simulink model "steady_state_model_verification"  (R2022b)
settings: Solver=VariableStepAuto  StartTime=0.0  StopTime=tmax  FixedStep=sample_time/10  RelTol=1e-3
values from neighbouring files (symbols this model uses):
  D = D_amp * exp(1i * angle(V_required))    [custom_control.m]    (also in steady_state_model_verification_script.m = D_amp .* exp(1i*D_phase))
  driving_voltage = 48    [sim_params.m]
  k = 0.1    [sim_params.m]    (also in steady_state_model_verification_script.m = k_vals(i))
  max_current = 150    [sim_params.m]
  phase_nbits = 16    [sim_params.m]
  R1 = 0.26    [sim_params.m]
  R2 = 0.26    [sim_params.m]
  relative_deadtime = deadtime / (0.5/fc)    (= 0.2164375)    [sim_params.m]
  sample_time = 1/(fc*samples_per_period)    (= 2.25599191452e-07)    [sim_params.m]
  samples_per_period = 32*4    (= 128)    [sim_params.m]
libraries: simulink x10, fl_lib x6, nesl_utility x5, ee_lib x4
settings Model: Creator=knasr  LastModifiedBy=nasrk
settings DebuggingCC: ParameterPrecisionLossMsg=none

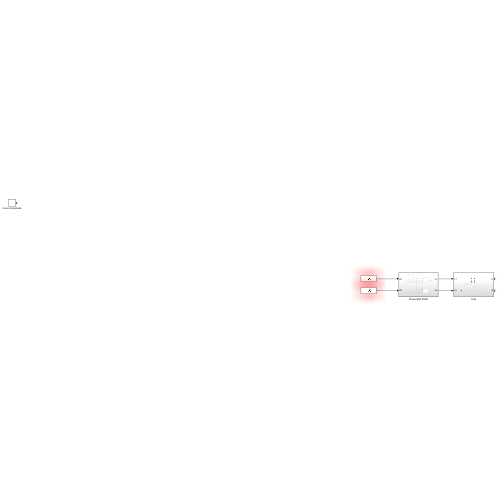
[thumbnail: Simulink's stored preview of the top-level diagram]
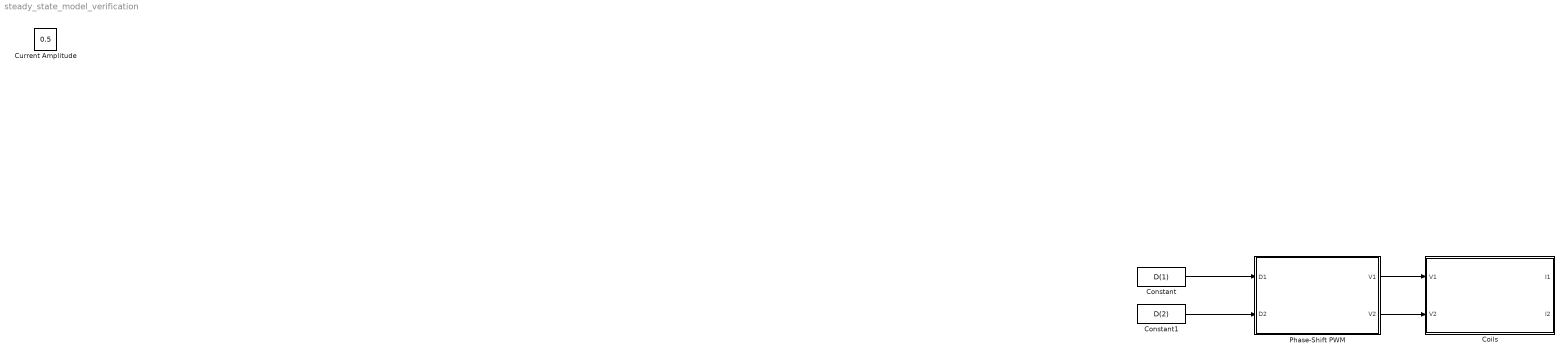
== system steady_state_model_verification ==
  Coils : Subsystem
  Constant : Constant  Value=D(1)  SampleTime=sample_time
  Constant1 : Constant  Value=D(2)  SampleTime=sample_time
  Current Amplitude : Constant  Value=0.5
  Phase-Shift PWM : Subsystem
  wires:
  Phase-Shift PWM/1(V1) -> Coils/1(V1)
  Phase-Shift PWM/2(V2) -> Coils/2(V2)
  Constant/1 -> Phase-Shift PWM/1(D1)
  Constant1/1 -> Phase-Shift PWM/2(D2)

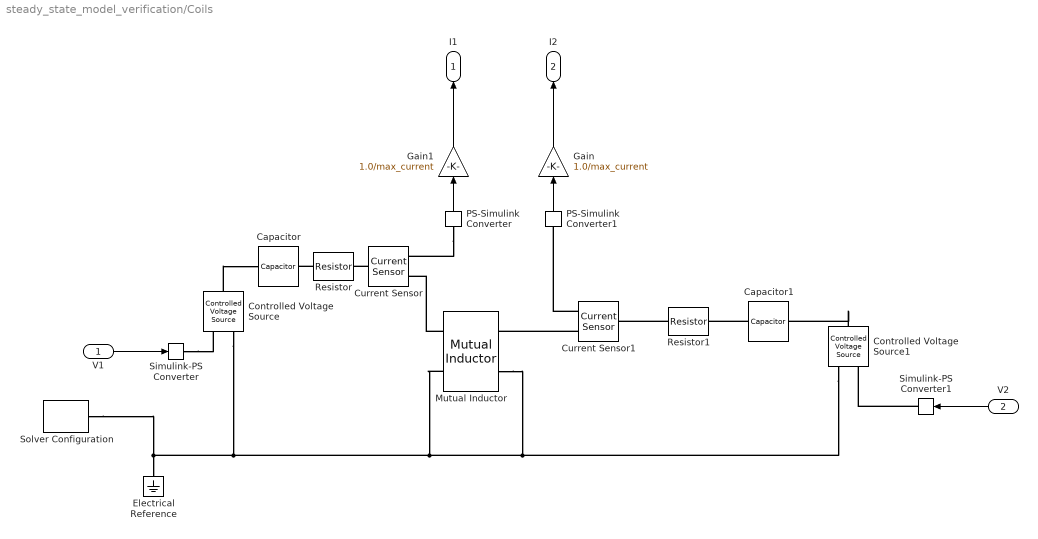
== system steady_state_model_verification/Coils ==
  V1 : Inport
  V2 : Inport  Port=2
  Capacitor : ee_lib/Passive/Capacitor  cap_option=0  c=C1 F  Cvec=[1e-05, 1e-06] F  Vvec=[0, 10] V  CV_table_symmetry=1  f_vec=[1, 10] kHz  DFext_vec=[.8, 1.2]  enable_C_tol=0  C_tol=5  tol_distribution=1  nSigma=4  r=1e-6 Ohm  g=0 1/Ohm  averaging_period=0 s  enable_operating_limits=0  operating_limit_action=2  max_working_voltage_range=[-25, 25] V  power_rating=1 W  enable_faults=0  fault_action=1  Cscale_faulted=100  R_faulted=1e-3 Ohm  G_faulted=0 1/Ohm  tau_fault=1e-3 s  enable_temporal_fault=0  t_fault=1 s  enable_behavioral_fault=0  max_permissible_voltage_range=[-100, 100] V  t_fail_on_voltage=1 s  i_specify=off  i_priority=None  i=0 A  i_nominal_specify=off  i_nominal_unit=A  i_nominal_value=1  v_specify=off  v_priority=None  v=0 V  v_nominal_specify=off  v_nominal_unit=V  v_nominal_value=1  vc_specify=off  vc_priority=High  vc=0 V  vc_nominal_specify=off  vc_nominal_unit=V  vc_nominal_value=1
  Capacitor1 : ee_lib/Passive/Capacitor  cap_option=0  c=C2 F  Cvec=[1e-05, 1e-06] F  Vvec=[0, 10] V  CV_table_symmetry=1  f_vec=[1, 10] kHz  DFext_vec=[.8, 1.2]  enable_C_tol=0  C_tol=5  tol_distribution=1  nSigma=4  r=1e-6 Ohm  g=0 1/Ohm  averaging_period=0 s  enable_operating_limits=0  operating_limit_action=2  max_working_voltage_range=[-25, 25] V  power_rating=1 W  enable_faults=0  fault_action=1  Cscale_faulted=100  R_faulted=1e-3 Ohm  G_faulted=0 1/Ohm  tau_fault=1e-3 s  enable_temporal_fault=0  t_fault=1 s  enable_behavioral_fault=0  max_permissible_voltage_range=[-100, 100] V  t_fail_on_voltage=1 s  i_specify=off  i_priority=None  i=0 A  i_nominal_specify=off  i_nominal_unit=A  i_nominal_value=1  v_specify=off  v_priority=None  v=0 V  v_nominal_specify=off  v_nominal_unit=V  v_nominal_value=1  vc_specify=off  vc_priority=High  vc=0 V  vc_nominal_specify=off  vc_nominal_unit=V  vc_nominal_value=1
  Controlled Voltage Source : fl_lib/Electrical/Electrical Sources/Controlled Voltage Source
  Controlled Voltage Source1 : fl_lib/Electrical/Electrical Sources/Controlled Voltage Source
  Current Sensor : fl_lib/Electrical/Electrical Sensors/Current Sensor
  Current Sensor1 : fl_lib/Electrical/Electrical Sensors/Current Sensor
  Electrical Reference : fl_lib/Electrical/Electrical Elements/Electrical Reference
  Gain : Gain  Gain=1.0/max_current
  Gain1 : Gain  Gain=1.0/max_current
  Mutual Inductor : fl_lib/Electrical/Electrical Elements/Mutual Inductor  L1=L1 H  L2=L2 H  k=k  i1_specify=off  i1_priority=High  i1=0 A  i1_nominal_specify=off  i1_nominal_unit=A  i1_nominal_value=1  i2_specify=off  i2_priority=High  i2=0 A  i2_nominal_specify=off  i2_nominal_unit=A  i2_nominal_value=1  v1_specify=off  v1_priority=None  v1=0 V  v1_nominal_specify=off  v1_nominal_unit=V  v1_nominal_value=1  v2_specify=off  v2_priority=None  v2=0 V  v2_nominal_specify=off  v2_nominal_unit=V  v2_nominal_value=1
      settings: InternalSimscapePortConfiguration="{\"Bottom\":[],\"Left\":[{\"id\":\"p1\",\"label\":\"1+\",\"type\":\"foundation.electrical.electrical\"},{\"id\":\"n1\",\"label\":\"1-\",\"type\":\"foundation.electrical.electrical\"}],\"Right\":[{\"id\":\"p2\",\"label\":\"2+\",\"type\":\"foundation.electrical.electrical\"},{\"id\":\"n2\",\"label\":\"2-\",\"type\":\"foundation.electrical.electrical\"}],\"Top\":[]}"
  PS-Simulink Converter : nesl_utility/PS-Simulink Converter  PhysicalDomain=network_engine_domain  SubClassName=ps_output  LeftPortType=input  RightPortType=output  PseudoPeriodic=off  Frequencies=[]  VectorFormat=inherit  Unit=inherit  AffineConversion=off
  PS-Simulink Converter1 : nesl_utility/PS-Simulink Converter  PhysicalDomain=network_engine_domain  SubClassName=ps_output  LeftPortType=input  RightPortType=output  PseudoPeriodic=off  Frequencies=[]  VectorFormat=inherit  Unit=inherit  AffineConversion=off
  Resistor : ee_lib/Passive/Resistor  R=R1 Ohm  enable_R_tol=0  R_tol=5  tol_distribution=1  nSigma=4  enable_operating_limits=0  operating_limit_action=2  max_working_voltage=100 V  power_rating=1 W  enable_faults=0  fault_action=1  R_faulted=inf Ohm  enable_temporal_fault=0  t_fault=1 s  enable_behavioral_fault=0  max_permissible_current=1 A  t_fail_on_current=1 s  noise_mode=0  sample_time=1e-3 s  repeatability=1  auto_seed=545404223  user_seed=0  Tdevice=25 degC  power_derating_T1=70 degC  power_derating_T2=155 degC  operating_temperature_range_vec=[-50, 150] degC  alpha=3.93e-3 1/K  Tmeas=25 degC  thermal_mass=100 J/K  temperature_specify=off  temperature_priority=High  temperature=298.15 K  temperature_nominal_specify=off  temperature_nominal_unit=K  temperature_nominal_value=1
  Resistor1 : ee_lib/Passive/Resistor  R=R2 Ohm  enable_R_tol=0  R_tol=5  tol_distribution=1  nSigma=4  enable_operating_limits=0  operating_limit_action=2  max_working_voltage=100 V  power_rating=1 W  enable_faults=0  fault_action=1  R_faulted=inf Ohm  enable_temporal_fault=0  t_fault=1 s  enable_behavioral_fault=0  max_permissible_current=1 A  t_fail_on_current=1 s  noise_mode=0  sample_time=1e-3 s  repeatability=1  auto_seed=3922919431  user_seed=0  Tdevice=25 degC  power_derating_T1=70 degC  power_derating_T2=155 degC  operating_temperature_range_vec=[-50, 150] degC  alpha=3.93e-3 1/K  Tmeas=25 degC  thermal_mass=100 J/K  temperature_specify=off  temperature_priority=High  temperature=298.15 K  temperature_nominal_specify=off  temperature_nominal_unit=K  temperature_nominal_value=1
  Simulink-PS Converter : nesl_utility/Simulink-PS Converter  PhysicalDomain=network_engine_domain  SubClassName=ps_input  LeftPortType=input  RightPortType=output  PseudoPeriodic=off  Frequencies=[]  NoiseDistribution=none  NoiseParameters=[]  Unit=1  AffineConversion=off  FilteringAndDerivatives=provide  SimscapeFilterOrder=1  InputFilterTimeConstant=0.001  UdotUserProvided=0
  Simulink-PS Converter1 : nesl_utility/Simulink-PS Converter  PhysicalDomain=network_engine_domain  SubClassName=ps_input  LeftPortType=input  RightPortType=output  PseudoPeriodic=off  Frequencies=[]  NoiseDistribution=none  NoiseParameters=[]  Unit=1  AffineConversion=off  FilteringAndDerivatives=provide  SimscapeFilterOrder=1  InputFilterTimeConstant=0.001  UdotUserProvided=0
  Solver Configuration : nesl_utility/Solver Configuration  PhysicalDomain=network_engine_domain  SubClassName=solver  LeftPortType=input  RightPortType=generic  Tones=[]  Harmonics=[]  SimulateNoise=off  Profile=off  UseLocalSampling=off  EnableSwitchedLinearOptims=on  FrequencyDomain=off  UseCCode=off  RelTol=0.001  AbsTol=1e-06  MinStep=1e-09  ToWorkspace=off  RevertToSquareIcSolve=off  NumHomotopyIterations=100  PhasorMode=off  PhasorModeNumHarmonics=1  ConsistencySolver=NEWTON_XTOL_AFTER_FTOL  IndexReductionMethod=DerivativeReplacement  DoDC=off  ResidualTolerance=1e-09  ConsistencyTolSource=GLOBAL  ConsistencyAbsTol=0.001  ConsistencyRelTol=0.001  ConsistencyTolFactor=0.001  UseLocalSolver=off  LocalSolverChoice=NE_BACKWARD_EULER_ADVANCER  ResolveIndetEquations=on  FunctionEvalNumThread=1  LocalSolverSampleTime=0.001  DoFixedCost=off  MaxNonlinIter=3  MaxModeIter=2  ComputeImpulses=off  ImpulseIterations=2  LinearAlgebra=auto  LinearAlgebraNumThread=0  EquationFormulation=NE_TIME_EF  DelaysMemoryBudget=1024  AutomaticFiltering=on  FilteringTimeConstant=0.001  PartitionStorageMethod=AS_NEEDED  PartitionMemoryBudget=1024  PartitionMethod=ROBUST
  I1 : Outport
  I2 : Outport  Port=2
  wires:
  V1/1 -> Simulink-PS Converter/1
  PS-Simulink Converter/1 -> Gain1/1
  V2/1 -> Simulink-PS Converter1/1
  PS-Simulink Converter1/1 -> Gain/1
  Gain/1 -> I2/1
  Gain1/1 -> I1/1
  connections:
  Mutual Inductor/RConn2 -- Mutual Inductor/LConn2 -- Solver Configuration/RConn1 -- Electrical Reference/LConn1 -- Controlled Voltage Source/RConn2 -- Controlled Voltage Source1/RConn2
  Resistor/LConn1 -- Capacitor/LConn1
  Current Sensor/LConn1 -- Resistor/RConn1
  Simulink-PS Converter/RConn1 -- Controlled Voltage Source/RConn1
  PS-Simulink Converter/LConn1 -- Current Sensor/RConn1
  Controlled Voltage Source/LConn1 -- Capacitor/RConn1
  Mutual Inductor/LConn1 -- Current Sensor/RConn2
  Capacitor1/RConn1 -- Resistor1/RConn1
  Simulink-PS Converter1/RConn1 -- Controlled Voltage Source1/RConn1
  Controlled Voltage Source1/LConn1 -- Capacitor1/LConn1
  Resistor1/LConn1 -- Current Sensor1/LConn1
  Current Sensor1/RConn2 -- Mutual Inductor/RConn1
  Current Sensor1/RConn1 -- PS-Simulink Converter1/LConn1

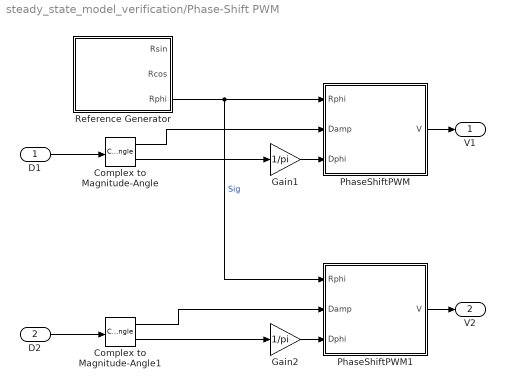
== system steady_state_model_verification/Phase-Shift PWM ==
  D1 : Inport
  D2 : Inport  Port=2
  Complex to Magnitude-Angle : ComplexToMagnitudeAngle
  Complex to Magnitude-Angle1 : ComplexToMagnitudeAngle
  Gain1 : Gain  Gain=1/pi
  Gain2 : Gain  Gain=1/pi
  PhaseShiftPWM : Subsystem
  PhaseShiftPWM1 : Subsystem
  Reference Generator : Subsystem
  V1 : Outport
  V2 : Outport  Port=2
  wires:
  D2/1 -> Complex to Magnitude-Angle1/1
  Complex to Magnitude-Angle/2 -> Gain1/1
  Complex to Magnitude-Angle1/2 -> Gain2/1
  Complex to Magnitude-Angle1/1 -> PhaseShiftPWM1/2(Damp)
  D1/1 -> Complex to Magnitude-Angle/1
  Gain1/1 -> PhaseShiftPWM/3(Dphi)
  Gain2/1 -> PhaseShiftPWM1/3(Dphi)
  Reference Generator/3(Rphi) -> PhaseShiftPWM1/1(Rphi), PhaseShiftPWM/1(Rphi)  "Sig"
  Complex to Magnitude-Angle/1 -> PhaseShiftPWM/2(Damp)
  PhaseShiftPWM/1(V) -> V1/1
  PhaseShiftPWM1/1(V) -> V2/1

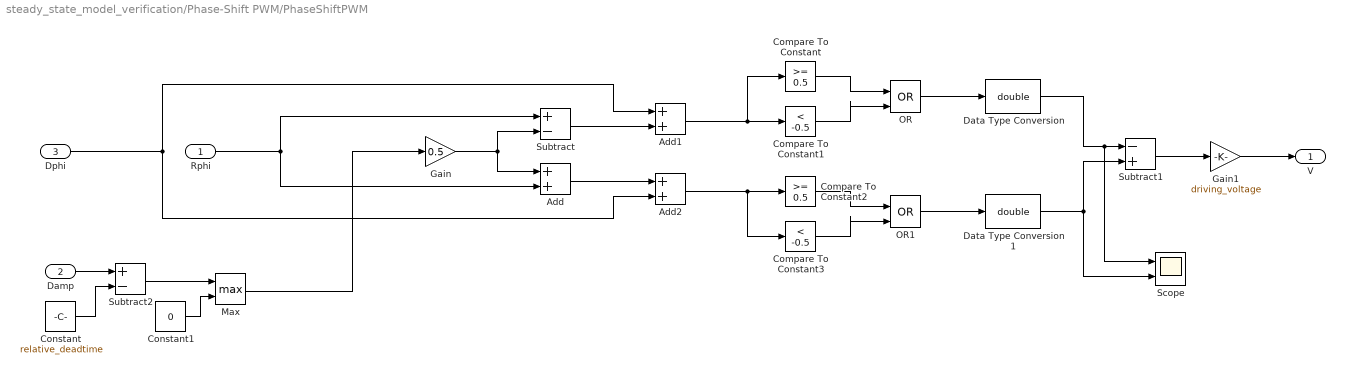
== system steady_state_model_verification/Phase-Shift PWM/PhaseShiftPWM ==
  Rphi : Inport
  Damp : Inport  Port=2
  Dphi : Inport  Port=3
  Add : Sum  AccumDataTypeStr=fixdt(1,phase_nbits,phase_nbits-1)  OutDataTypeStr=fixdt(1,phase_nbits,phase_nbits-1)
  Add1 : Sum  AccumDataTypeStr=fixdt(1,phase_nbits,phase_nbits-1)  OutDataTypeStr=fixdt(1,phase_nbits,phase_nbits-1)
  Add2 : Sum  AccumDataTypeStr=fixdt(1,phase_nbits,phase_nbits-1)  OutDataTypeStr=fixdt(1,phase_nbits,phase_nbits-1)
  Compare To Constant : simulink/Logic and Bit Operations/Compare To Constant  relop=>=  const=0.5  OutDataTypeStr=boolean
  Compare To Constant1 : simulink/Logic and Bit Operations/Compare To Constant  relop=<  const=-0.5  OutDataTypeStr=boolean
  Compare To Constant2 : simulink/Logic and Bit Operations/Compare To Constant  relop=>=  const=0.5  OutDataTypeStr=boolean
  Compare To Constant3 : simulink/Logic and Bit Operations/Compare To Constant  relop=<  const=-0.5  OutDataTypeStr=boolean
  Constant : Constant  Value=relative_deadtime
  Constant1 : Constant  Value=0
  Data Type Conversion : DataTypeConversion  OutDataTypeStr=double  SaturateOnIntegerOverflow=off  RndMeth=Floor
  Data Type Conversion1 : DataTypeConversion  OutDataTypeStr=double  SaturateOnIntegerOverflow=off  RndMeth=Floor
  Gain : Gain  Gain=0.5  ParamDataTypeStr=fixdt(1,phase_nbits,phase_nbits-1)  OutDataTypeStr=fixdt(1,phase_nbits,phase_nbits-1)
  Gain1 : Gain  Gain=driving_voltage
  Max : MinMax  Function=max  Inputs=2
  OR : Logic  Operator=OR  IconShape=distinctive  AllPortsSameDT=off  OutDataTypeStr=boolean
  OR1 : Logic  Operator=OR  IconShape=distinctive  AllPortsSameDT=off  OutDataTypeStr=boolean
  Scope : Scope  NumInputPorts=2
  Subtract : Sum  Inputs=+-  AccumDataTypeStr=fixdt(1,phase_nbits,phase_nbits-1)  OutDataTypeStr=fixdt(1,phase_nbits,phase_nbits-1)
  Subtract1 : Sum  Inputs=-+
  Subtract2 : Sum  Inputs=+-
  V : Outport
  wires:
  Gain/1 -> Add/1, Subtract/2
  Rphi/1 -> Subtract/1, Add/2
  Subtract/1 -> Add1/2
  Add/1 -> Add2/1
  Dphi/1 -> Add1/1, Add2/2
  Add1/1 -> Compare To Constant/1, Compare To Constant1/1
  Compare To Constant/1 -> OR/1
  Compare To Constant1/1 -> OR/2
  Compare To Constant2/1 -> OR1/1
  Compare To Constant3/1 -> OR1/2
  Add2/1 -> Compare To Constant3/1, Compare To Constant2/1
  OR1/1 -> Data Type Conversion1/1
  OR/1 -> Data Type Conversion/1
  Data Type Conversion/1 -> Scope/1, Subtract1/1
  Data Type Conversion1/1 -> Subtract1/2, Scope/2
  Subtract1/1 -> Gain1/1
  Gain1/1 -> V/1
  Damp/1 -> Subtract2/1
  Constant/1 -> Subtract2/2
  Subtract2/1 -> Max/1
  Constant1/1 -> Max/2
  Max/1 -> Gain/1

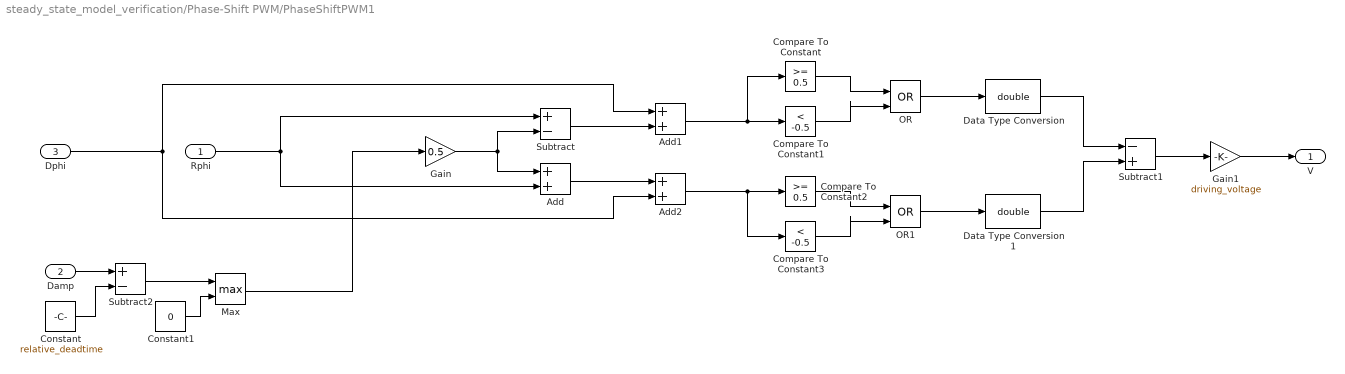
== system steady_state_model_verification/Phase-Shift PWM/PhaseShiftPWM1 ==
  Rphi : Inport
  Damp : Inport  Port=2
  Dphi : Inport  Port=3
  Add : Sum  AccumDataTypeStr=fixdt(1,phase_nbits,phase_nbits-1)  OutDataTypeStr=fixdt(1,phase_nbits,phase_nbits-1)
  Add1 : Sum  AccumDataTypeStr=fixdt(1,phase_nbits,phase_nbits-1)  OutDataTypeStr=fixdt(1,phase_nbits,phase_nbits-1)
  Add2 : Sum  AccumDataTypeStr=fixdt(1,phase_nbits,phase_nbits-1)  OutDataTypeStr=fixdt(1,phase_nbits,phase_nbits-1)
  Compare To Constant : simulink/Logic and Bit Operations/Compare To Constant  relop=>=  const=0.5  OutDataTypeStr=boolean
  Compare To Constant1 : simulink/Logic and Bit Operations/Compare To Constant  relop=<  const=-0.5  OutDataTypeStr=boolean
  Compare To Constant2 : simulink/Logic and Bit Operations/Compare To Constant  relop=>=  const=0.5  OutDataTypeStr=boolean
  Compare To Constant3 : simulink/Logic and Bit Operations/Compare To Constant  relop=<  const=-0.5  OutDataTypeStr=boolean
  Constant : Constant  Value=relative_deadtime
  Constant1 : Constant  Value=0
  Data Type Conversion : DataTypeConversion  OutDataTypeStr=double  SaturateOnIntegerOverflow=off  RndMeth=Floor
  Data Type Conversion1 : DataTypeConversion  OutDataTypeStr=double  SaturateOnIntegerOverflow=off  RndMeth=Floor
  Gain : Gain  Gain=0.5  ParamDataTypeStr=fixdt(1,phase_nbits,phase_nbits-1)  OutDataTypeStr=fixdt(1,phase_nbits,phase_nbits-1)
  Gain1 : Gain  Gain=driving_voltage
  Max : MinMax  Function=max  Inputs=2
  OR : Logic  Operator=OR  IconShape=distinctive  AllPortsSameDT=off  OutDataTypeStr=boolean
  OR1 : Logic  Operator=OR  IconShape=distinctive  AllPortsSameDT=off  OutDataTypeStr=boolean
  Subtract : Sum  Inputs=+-  AccumDataTypeStr=fixdt(1,phase_nbits,phase_nbits-1)  OutDataTypeStr=fixdt(1,phase_nbits,phase_nbits-1)
  Subtract1 : Sum  Inputs=-+
  Subtract2 : Sum  Inputs=+-
  V : Outport
  wires:
  Gain/1 -> Add/1, Subtract/2
  Rphi/1 -> Subtract/1, Add/2
  Subtract/1 -> Add1/2
  Add/1 -> Add2/1
  Dphi/1 -> Add1/1, Add2/2
  Add1/1 -> Compare To Constant/1, Compare To Constant1/1
  Compare To Constant/1 -> OR/1
  Compare To Constant1/1 -> OR/2
  Compare To Constant2/1 -> OR1/1
  Compare To Constant3/1 -> OR1/2
  Add2/1 -> Compare To Constant3/1, Compare To Constant2/1
  OR1/1 -> Data Type Conversion1/1
  OR/1 -> Data Type Conversion/1
  Data Type Conversion/1 -> Subtract1/1
  Data Type Conversion1/1 -> Subtract1/2
  Subtract1/1 -> Gain1/1
  Gain1/1 -> V/1
  Damp/1 -> Subtract2/1
  Constant/1 -> Subtract2/2
  Subtract2/1 -> Max/1
  Constant1/1 -> Max/2
  Max/1 -> Gain/1

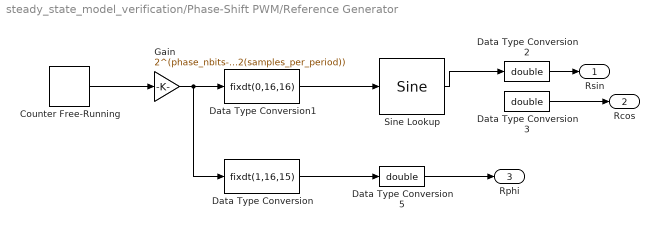
== system steady_state_model_verification/Phase-Shift PWM/Reference Generator ==
  Counter Free-Running : simulink/Sources/Counter Free-Running  NumBits=log2(samples_per_period)  tsamp=sample_time
  Data Type Conversion : DataTypeConversion  OutDataTypeStr=fixdt(1,16,15)  ConvertRealWorld=Stored Integer (SI)  SaturateOnIntegerOverflow=off  RndMeth=Floor
  Data Type Conversion1 : DataTypeConversion  OutDataTypeStr=fixdt(0,16,16)  ConvertRealWorld=Stored Integer (SI)  SaturateOnIntegerOverflow=off  RndMeth=Floor
  Data Type Conversion2 : DataTypeConversion  OutDataTypeStr=double  SaturateOnIntegerOverflow=off  RndMeth=Floor
  Data Type Conversion3 : DataTypeConversion  OutDataTypeStr=double  SaturateOnIntegerOverflow=off  RndMeth=Floor
  Data Type Conversion5 : DataTypeConversion  OutDataTypeStr=double  SaturateOnIntegerOverflow=off  RndMeth=Floor
  Gain : Gain  Gain=2^(phase_nbits-log2(samples_per_period))  OutDataTypeStr=uint16
  Sine Lookup : simulink/Lookup Tables/Sine  Formula=sin(2*pi*u) and cos(2*pi*u)  NumDataPoints=2^(phase_nbits-2)+1  OutputWordLength=phase_nbits  InternalRulePriority=Speed
      settings: LibrarySourceBlock=|
      | simulink/Quick Insert/Lookup
      | Tables/Sine Lookup
  Rsin : Outport
  Rcos : Outport  Port=2
  Rphi : Outport  Port=3
  wires:
  Counter Free-Running/1 -> Gain/1
  Gain/1 -> Data Type Conversion/1, Data Type Conversion1/1
  Data Type Conversion1/1 -> Sine Lookup/1
  Sine Lookup/1 -> Data Type Conversion2/1
  ? -> Data Type Conversion3/1
  Data Type Conversion2/1 -> Rsin/1
  Data Type Conversion3/1 -> Rcos/1
  Data Type Conversion/1 -> Data Type Conversion5/1
  Data Type Conversion5/1 -> Rphi/1
